simulink model "Speedmeter"  (R2019b)
settings: Solver=FixedStepDiscrete  StartTime=0.0  StopTime=5  FixedStep=0.01  RelTol=1e-3
undefined symbols (not defined in the file or in its folder): Const16_0, Const16_2, Const16_210, Const16_340, Const16_350, Const16_4, Const8_0, Const8_1, Const8_2, Const8_4, ConstFL_00879, ConstFL_01, ConstFL_03516, ConstFL_1_6093, STEP_TIME
libraries: simulink x1
(part 1 of 2)
Description:
  | Integrated model for MBD SWC SpeedMeter
settings Model: DataTypeOverride=Single  ModifiedByFormat=TATA ELXSI LTD  Creator=TATA ELXSI LTD  LastModifiedBy=TATA ELXSI LTD
settings ConfigSet: Description=Test1
settings DataIOCC: LimitDataPoints=on  SaveFormat=StructureWithTime  ReturnWorkspaceOutputs=off
settings OptimizationCC: LifeSpan=inf
settings DebuggingCC: UnderspecifiedInitializationDetection=Classic  MergeDetectMultiDrivingBlocksExec=none  SolverPrmCheckMsg=warning  InheritedTsInSrcMsg=none  ParameterPrecisionLossMsg=none  FcnCallInpInsideContextMsg=warning  StateNameClashWarn=warning  SFUnexpectedBacktrackingDiag=warning  SFNoUnconditionalDefaultTransitionDiag=warning  SFExecutionAtInitializationDiag=none
settings HardwareCC: ProdBitPerPointer=32  ProdBitPerSizeT=32  ProdBitPerPtrDiffT=32  ProdLargestAtomicFloat=None  ProdWordSize=32  ProdHWDeviceType=Generic->32-bit x86 compatible
settings ModelReferenceCC: PropagateSignalLabelsOutOfModel=off
settings RTWCC: Description=Generic Real-Time Target
settings CodeAppCC: StateflowObjectComments=on
settings GRTTargetCC: TargetLangStandard=C89/C90 (ANSI)  CombineOutputUpdateFcns=off  GRTInterface=on
settings ConfigComp: DVMaxTestCaseSteps=500  DVTestSuiteOptimization=CombinedObjectives (Nonlinear Extended)  DVDetectDeadLogic=on  DVDetectActiveLogic=on  DVDetectOutOfBounds=on

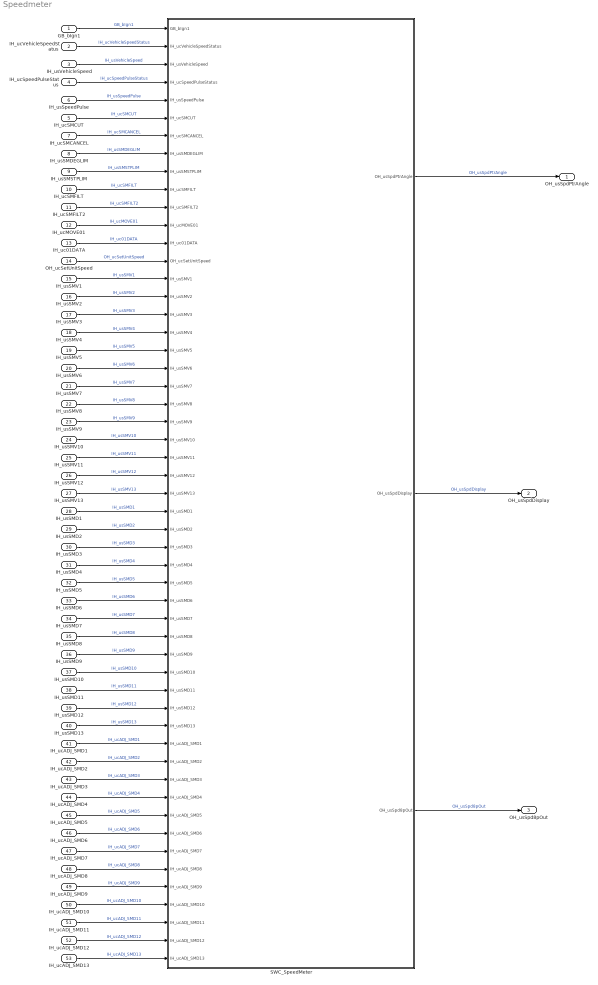
== system Speedmeter ==
  GB_bIgn1 : Inport  OutMin=0  OutMax=1  OutDataTypeStr=uint8  SampleTime=STEP_TIME
  IH_ucVehicleSpeedStatus : Inport  Port=2  OutMin=0  OutMax=3  OutDataTypeStr=fixdt(0,8,1,0)  SampleTime=STEP_TIME
  IH_usVehicleSpeed : Inport  Port=3  OutMin=0  OutMax=655.35  OutDataTypeStr=fixdt(0,16,0.01,0)  SampleTime=STEP_TIME
  IH_ucSpeedPulseStatus : Inport  Port=4  OutMin=0  OutMax=3  OutDataTypeStr=fixdt(0,8,1,0)  SampleTime=STEP_TIME
  IH_ucSMCUT : Inport  Port=5  OutMin=0  OutMax=3  OutDataTypeStr=fixdt(0,8,1,0)  SampleTime=STEP_TIME
  IH_usSpeedPulse : Inport  Port=6  OutMin=0  OutMax=655.35  OutDataTypeStr=fixdt(0,16,0.01,0)  SampleTime=STEP_TIME
  IH_ucSMCANCEL : Inport  Port=7  OutMin=0  OutMax=10.8996  OutDataTypeStr=fixdt(0,8,0.3516,0)  SampleTime=STEP_TIME
  IH_usSMDEGLIM : Inport  Port=8  OutMin=0  OutMax=359.6868  OutDataTypeStr=fixdt(0,16,0.3516,0)  SampleTime=STEP_TIME
  IH_usSMSTPLIM : Inport  Port=9  OutMin=0  OutMax=5.5377  OutDataTypeStr=fixdt(0,16,0.0879,0)  SampleTime=STEP_TIME
  IH_ucSMFILT : Inport  Port=10  OutMin=0  OutMax=7  OutDataTypeStr=fixdt(0,8,1,0)  SampleTime=STEP_TIME
  IH_ucSMFILT2 : Inport  Port=11  OutMin=0  OutMax=7  OutDataTypeStr=fixdt(0,8,1,0)  SampleTime=STEP_TIME
  IH_ucMOVE01 : Inport  Port=12  OutMin=0  OutMax=3  OutDataTypeStr=fixdt(0,8,1,0)  SampleTime=STEP_TIME
  IH_uc01DATA : Inport  Port=13  OutMin=0  OutMax=1  OutDataTypeStr=fixdt(0,8,1,0)  SampleTime=STEP_TIME
  OH_ucSetUnitSpeed : Inport  Port=14  OutMin=0  OutMax=1  OutDataTypeStr=fixdt(0,8,1,0)  SampleTime=STEP_TIME
  IH_usSMV1 : Inport  Port=15  OutMin=0  OutMax=409.5  OutDataTypeStr=fixdt(0,16,0.1,0)  SampleTime=STEP_TIME
  IH_usSMV2 : Inport  Port=16  OutMin=0  OutMax=409.5  OutDataTypeStr=fixdt(0,16,0.1,0)  SampleTime=STEP_TIME
  IH_usSMV3 : Inport  Port=17  OutMin=0  OutMax=409.5  OutDataTypeStr=fixdt(0,16,0.1,0)  SampleTime=STEP_TIME
  IH_usSMV4 : Inport  Port=18  OutMin=0  OutMax=409.5  OutDataTypeStr=fixdt(0,16,0.1,0)  SampleTime=STEP_TIME
  IH_usSMV5 : Inport  Port=19  OutMin=0  OutMax=409.5  OutDataTypeStr=fixdt(0,16,0.1,0)  SampleTime=STEP_TIME
  IH_usSMV6 : Inport  Port=20  OutMin=0  OutMax=409.5  OutDataTypeStr=fixdt(0,16,0.1,0)  SampleTime=STEP_TIME
  IH_usSMV7 : Inport  Port=21  OutMin=0  OutMax=409.5  OutDataTypeStr=fixdt(0,16,0.1,0)  SampleTime=STEP_TIME
  IH_usSMV8 : Inport  Port=22  OutMin=0  OutMax=409.5  OutDataTypeStr=fixdt(0,16,0.1,0)  SampleTime=STEP_TIME
  IH_usSMV9 : Inport  Port=23  OutMin=0  OutMax=409.5  OutDataTypeStr=fixdt(0,16,0.1,0)  SampleTime=STEP_TIME
  IH_usSMV10 : Inport  Port=24  OutMin=0  OutMax=409.5  OutDataTypeStr=fixdt(0,16,0.1,0)  SampleTime=STEP_TIME
  IH_usSMV11 : Inport  Port=25  OutMin=0  OutMax=409.5  OutDataTypeStr=fixdt(0,16,0.1,0)  SampleTime=STEP_TIME
  IH_usSMV12 : Inport  Port=26  OutMin=0  OutMax=409.5  OutDataTypeStr=fixdt(0,16,0.1,0)  SampleTime=STEP_TIME
  IH_usSMV13 : Inport  Port=27  OutMin=0  OutMax=409.5  OutDataTypeStr=fixdt(0,16,0.1,0)  SampleTime=STEP_TIME
  IH_usSMD1 : Inport  Port=28  OutMin=0  OutMax=359.9505  OutDataTypeStr=fixdt(0,16,0.0879,0)  SampleTime=STEP_TIME
  IH_usSMD2 : Inport  Port=29  OutMin=0  OutMax=359.9505  OutDataTypeStr=fixdt(0,16,0.0879,0)  SampleTime=STEP_TIME
  IH_usSMD3 : Inport  Port=30  OutMin=0  OutMax=359.9505  OutDataTypeStr=fixdt(0,16,0.0879,0)  SampleTime=STEP_TIME
  IH_usSMD4 : Inport  Port=31  OutMin=0  OutMax=359.9505  OutDataTypeStr=fixdt(0,16,0.0879,0)  SampleTime=STEP_TIME
  IH_usSMD5 : Inport  Port=32  OutMin=0  OutMax=359.9505  OutDataTypeStr=fixdt(0,16,0.0879,0)  SampleTime=STEP_TIME
  IH_usSMD6 : Inport  Port=33  OutMin=0  OutMax=359.9505  OutDataTypeStr=fixdt(0,16,0.0879,0)  SampleTime=STEP_TIME
  IH_usSMD7 : Inport  Port=34  OutMin=0  OutMax=359.9505  OutDataTypeStr=fixdt(0,16,0.0879,0)  SampleTime=STEP_TIME
  IH_usSMD8 : Inport  Port=35  OutMin=0  OutMax=359.9505  OutDataTypeStr=fixdt(0,16,0.0879,0)  SampleTime=STEP_TIME
  IH_usSMD9 : Inport  Port=36  OutMin=0  OutMax=359.9505  OutDataTypeStr=fixdt(0,16,0.0879,0)  SampleTime=STEP_TIME
  IH_usSMD10 : Inport  Port=37  OutMin=0  OutMax=359.9505  OutDataTypeStr=fixdt(0,16,0.0879,0)  SampleTime=STEP_TIME
  IH_usSMD11 : Inport  Port=38  OutMin=0  OutMax=359.9505  OutDataTypeStr=fixdt(0,16,0.0879,0)  SampleTime=STEP_TIME
  IH_usSMD12 : Inport  Port=39  OutMin=0  OutMax=359.9505  OutDataTypeStr=fixdt(0,16,0.0879,0)  SampleTime=STEP_TIME
  IH_usSMD13 : Inport  Port=40  OutMin=0  OutMax=359.9505  OutDataTypeStr=fixdt(0,16,0.0879,0)  SampleTime=STEP_TIME
  IH_ucADJ_SMD1 : Inport  Port=41  OutMin=0  OutMax=22.4145  OutDataTypeStr=fixdt(0,8,0.0879,0)  SampleTime=STEP_TIME
  IH_ucADJ_SMD2 : Inport  Port=42  OutMin=0  OutMax=22.4145  OutDataTypeStr=fixdt(0,8,0.0879,0)  SampleTime=STEP_TIME
  IH_ucADJ_SMD3 : Inport  Port=43  OutMin=0  OutMax=22.4145  OutDataTypeStr=fixdt(0,8,0.0879,0)  SampleTime=STEP_TIME
  IH_ucADJ_SMD4 : Inport  Port=44  OutMin=0  OutMax=22.4145  OutDataTypeStr=fixdt(0,8,0.0879,0)  SampleTime=STEP_TIME
  IH_ucADJ_SMD5 : Inport  Port=45  OutMin=0  OutMax=22.4145  OutDataTypeStr=fixdt(0,8,0.0879,0)  SampleTime=STEP_TIME
  IH_ucADJ_SMD6 : Inport  Port=46  OutMin=0  OutMax=22.4145  OutDataTypeStr=fixdt(0,8,0.0879,0)  SampleTime=STEP_TIME
  IH_ucADJ_SMD7 : Inport  Port=47  OutMin=0  OutMax=22.4145  OutDataTypeStr=fixdt(0,8,0.0879,0)  SampleTime=STEP_TIME
  IH_ucADJ_SMD8 : Inport  Port=48  OutMin=0  OutMax=22.4145  OutDataTypeStr=fixdt(0,8,0.0879,0)  SampleTime=STEP_TIME
  IH_ucADJ_SMD9 : Inport  Port=49  OutMin=0  OutMax=22.4145  OutDataTypeStr=fixdt(0,8,0.0879,0)  SampleTime=STEP_TIME
  IH_ucADJ_SMD10 : Inport  Port=50  OutMin=0  OutMax=22.4145  OutDataTypeStr=fixdt(0,8,0.0879,0)  SampleTime=STEP_TIME
  IH_ucADJ_SMD11 : Inport  Port=51  OutMin=0  OutMax=22.4145  OutDataTypeStr=fixdt(0,8,0.0879,0)  SampleTime=STEP_TIME
  IH_ucADJ_SMD12 : Inport  Port=52  OutMin=0  OutMax=22.4145  OutDataTypeStr=fixdt(0,8,0.0879,0)  SampleTime=STEP_TIME
  IH_ucADJ_SMD13 : Inport  Port=53  OutMin=0  OutMax=22.4145  OutDataTypeStr=fixdt(0,8,0.0879,0)  SampleTime=STEP_TIME
  SWC_SpeedMeter : Subsystem  LoadFcn=set_param('Speedmeter', 'DataTypeOverride','Single')  TreatAsAtomicUnit=on
  OH_usSpdPtrAngle : Outport  OutMin=0  OutMax=4095  OutDataTypeStr=fixdt(0,16,0.0879,0)  SampleTime=STEP_TIME  VectorParamsAs1DForOutWhenUnconnected=off
  OH_usSpdDisplay : Outport  Port=2  OutDataTypeStr=fixdt(0,16,1,0)  SampleTime=STEP_TIME  VectorParamsAs1DForOutWhenUnconnected=off
  OH_usSpd8pOut : Outport  Port=3  OutMin=0  OutMax=655.34  OutDataTypeStr=fixdt(0,16,0.01,0)  SampleTime=STEP_TIME  VectorParamsAs1DForOutWhenUnconnected=off
  wires:
  IH_ucVehicleSpeedStatus/1 -> SWC_SpeedMeter/2(IH_ucVehicleSpeedStatus)  "IH_ucVehicleSpeedStatus"
  IH_usSMV12/1 -> SWC_SpeedMeter/26(IH_usSMV12)  "IH_usSMV12"
  GB_bIgn1/1 -> SWC_SpeedMeter/1(GB_bIgn1)  "GB_bIgn1"
  IH_ucADJ_SMD6/1 -> SWC_SpeedMeter/46(IH_ucADJ_SMD6)  "IH_ucADJ_SMD6"
  IH_ucADJ_SMD7/1 -> SWC_SpeedMeter/47(IH_ucADJ_SMD7)  "IH_ucADJ_SMD7"
  IH_uc01DATA/1 -> SWC_SpeedMeter/13(IH_uc01DATA)  "IH_uc01DATA"
  IH_ucADJ_SMD12/1 -> SWC_SpeedMeter/52(IH_ucADJ_SMD12)  "IH_ucADJ_SMD12"
  IH_ucADJ_SMD13/1 -> SWC_SpeedMeter/53(IH_ucADJ_SMD13)  "IH_ucADJ_SMD13"
  IH_usVehicleSpeed/1 -> SWC_SpeedMeter/3(IH_usVehicleSpeed)  "IH_usVehicleSpeed"
  IH_ucADJ_SMD11/1 -> SWC_SpeedMeter/51(IH_ucADJ_SMD11)  "IH_ucADJ_SMD11"
  IH_ucADJ_SMD8/1 -> SWC_SpeedMeter/48(IH_ucADJ_SMD8)  "IH_ucADJ_SMD8"
  IH_usSMD9/1 -> SWC_SpeedMeter/36(IH_usSMD9)  "IH_usSMD9"
  IH_usSMD11/1 -> SWC_SpeedMeter/38(IH_usSMD11)  "IH_usSMD11"
  IH_usSMV2/1 -> SWC_SpeedMeter/16(IH_usSMV2)  "IH_usSMV2"
  IH_ucADJ_SMD3/1 -> SWC_SpeedMeter/43(IH_ucADJ_SMD3)  "IH_ucADJ_SMD3"
  IH_usSMD10/1 -> SWC_SpeedMeter/37(IH_usSMD10)  "IH_usSMD10"
  IH_usSMD3/1 -> SWC_SpeedMeter/30(IH_usSMD3)  "IH_usSMD3"
  IH_usSMD13/1 -> SWC_SpeedMeter/40(IH_usSMD13)  "IH_usSMD13"
  OH_ucSetUnitSpeed/1 -> SWC_SpeedMeter/14(OH_ucSetUnitSpeed)  "OH_ucSetUnitSpeed"
  IH_usSMDEGLIM/1 -> SWC_SpeedMeter/8(IH_usSMDEGLIM)  "IH_usSMDEGLIM"
  IH_usSMV13/1 -> SWC_SpeedMeter/27(IH_usSMV13)  "IH_usSMV13"
  IH_usSpeedPulse/1 -> SWC_SpeedMeter/5(IH_usSpeedPulse)  "IH_usSpeedPulse"
  IH_ucADJ_SMD5/1 -> SWC_SpeedMeter/45(IH_ucADJ_SMD5)  "IH_ucADJ_SMD5"
  IH_usSMD5/1 -> SWC_SpeedMeter/32(IH_usSMD5)  "IH_usSMD5"
  IH_ucSMCUT/1 -> SWC_SpeedMeter/6(IH_ucSMCUT)  "IH_ucSMCUT"
  IH_ucSMFILT2/1 -> SWC_SpeedMeter/11(IH_ucSMFILT2)  "IH_ucSMFILT2"
  IH_ucADJ_SMD2/1 -> SWC_SpeedMeter/42(IH_ucADJ_SMD2)  "IH_ucADJ_SMD2"
  IH_usSMD2/1 -> SWC_SpeedMeter/29(IH_usSMD2)  "IH_usSMD2"
  IH_usSMV9/1 -> SWC_SpeedMeter/23(IH_usSMV9)  "IH_usSMV9"
  IH_usSMV8/1 -> SWC_SpeedMeter/22(IH_usSMV8)  "IH_usSMV8"
  IH_usSMD4/1 -> SWC_SpeedMeter/31(IH_usSMD4)  "IH_usSMD4"
  IH_ucSpeedPulseStatus/1 -> SWC_SpeedMeter/4(IH_ucSpeedPulseStatus)  "IH_ucSpeedPulseStatus"
  IH_usSMD6/1 -> SWC_SpeedMeter/33(IH_usSMD6)  "IH_usSMD6"
  IH_usSMV7/1 -> SWC_SpeedMeter/21(IH_usSMV7)  "IH_usSMV7"
  IH_ucADJ_SMD4/1 -> SWC_SpeedMeter/44(IH_ucADJ_SMD4)  "IH_ucADJ_SMD4"
  IH_usSMSTPLIM/1 -> SWC_SpeedMeter/9(IH_usSMSTPLIM)  "IH_usSMSTPLIM"
  IH_usSMD8/1 -> SWC_SpeedMeter/35(IH_usSMD8)  "IH_usSMD8"
  IH_ucADJ_SMD9/1 -> SWC_SpeedMeter/49(IH_ucADJ_SMD9)  "IH_ucADJ_SMD9"
  IH_usSMV5/1 -> SWC_SpeedMeter/19(IH_usSMV5)  "IH_usSMV5"
  IH_usSMD12/1 -> SWC_SpeedMeter/39(IH_usSMD12)  "IH_usSMD12"
  IH_ucSMFILT/1 -> SWC_SpeedMeter/10(IH_ucSMFILT)  "IH_ucSMFILT"
  IH_usSMD1/1 -> SWC_SpeedMeter/28(IH_usSMD1)  "IH_usSMD1"
  IH_usSMV10/1 -> SWC_SpeedMeter/24(IH_usSMV10)  "IH_usSMV10"
  IH_usSMV3/1 -> SWC_SpeedMeter/17(IH_usSMV3)  "IH_usSMV3"
  IH_ucMOVE01/1 -> SWC_SpeedMeter/12(IH_ucMOVE01)  "IH_ucMOVE01"
  IH_ucADJ_SMD10/1 -> SWC_SpeedMeter/50(IH_ucADJ_SMD10)  "IH_ucADJ_SMD10"
  IH_usSMV1/1 -> SWC_SpeedMeter/15(IH_usSMV1)  "IH_usSMV1"
  IH_usSMV4/1 -> SWC_SpeedMeter/18(IH_usSMV4)  "IH_usSMV4"
  IH_usSMV6/1 -> SWC_SpeedMeter/20(IH_usSMV6)  "IH_usSMV6"
  IH_usSMV11/1 -> SWC_SpeedMeter/25(IH_usSMV11)  "IH_usSMV11"
  IH_ucADJ_SMD1/1 -> SWC_SpeedMeter/41(IH_ucADJ_SMD1)  "IH_ucADJ_SMD1"
  IH_ucSMCANCEL/1 -> SWC_SpeedMeter/7(IH_ucSMCANCEL)  "IH_ucSMCANCEL"
  IH_usSMD7/1 -> SWC_SpeedMeter/34(IH_usSMD7)  "IH_usSMD7"
  SWC_SpeedMeter/3(OH_usSpd8pOut) -> OH_usSpd8pOut/1  "OH_usSpd8pOut"
  SWC_SpeedMeter/1(OH_usSpdPtrAngle) -> OH_usSpdPtrAngle/1  "OH_usSpdPtrAngle"
  SWC_SpeedMeter/2(OH_usSpdDisplay) -> OH_usSpdDisplay/1  "OH_usSpdDisplay"

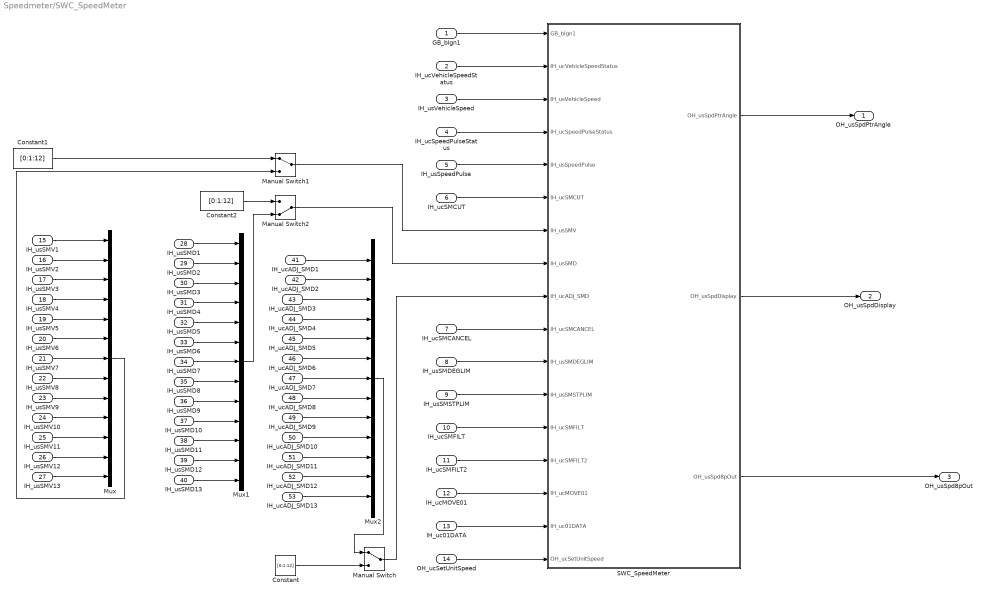
== system Speedmeter/SWC_SpeedMeter ==
  GB_bIgn1 : Inport  SampleTime=STEP_TIME
  IH_ucVehicleSpeedStatus : Inport  Port=2  OutDataTypeStr=fixdt(0,8,1,0)  SampleTime=STEP_TIME
  IH_usVehicleSpeed : Inport  Port=3  OutDataTypeStr=fixdt(0,16,0.01,0)  SampleTime=STEP_TIME
  IH_ucSpeedPulseStatus : Inport  Port=4  OutDataTypeStr=fixdt(0,8,1,0)  SampleTime=STEP_TIME
  IH_usSpeedPulse : Inport  Port=5  OutDataTypeStr=fixdt(0,16,0.01,0)  SampleTime=STEP_TIME
  IH_ucSMCUT : Inport  Port=6  OutDataTypeStr=fixdt(0,8,1,0)  SampleTime=STEP_TIME
  IH_ucSMCANCEL : Inport  Port=7  SampleTime=STEP_TIME
  IH_usSMDEGLIM : Inport  Port=8  SampleTime=STEP_TIME
  IH_usSMSTPLIM : Inport  Port=9  SampleTime=STEP_TIME
  IH_ucSMFILT : Inport  Port=10  OutDataTypeStr=fixdt(0,8,1,0)  SampleTime=STEP_TIME
  IH_ucSMFILT2 : Inport  Port=11  OutDataTypeStr=fixdt(0,8,1,0)  SampleTime=STEP_TIME
  IH_ucMOVE01 : Inport  Port=12  OutDataTypeStr=fixdt(0,8,1,0)  SampleTime=STEP_TIME
  IH_uc01DATA : Inport  Port=13  OutDataTypeStr=fixdt(0,8,1,0)  SampleTime=STEP_TIME
  OH_ucSetUnitSpeed : Inport  Port=14  OutDataTypeStr=fixdt(0,8,1,0)  SampleTime=STEP_TIME
  IH_usSMV1 : Inport  Port=15  SampleTime=STEP_TIME
  IH_usSMV2 : Inport  Port=16  SampleTime=STEP_TIME
  IH_usSMV3 : Inport  Port=17  SampleTime=STEP_TIME
  IH_usSMV4 : Inport  Port=18  SampleTime=STEP_TIME
  IH_usSMV5 : Inport  Port=19  SampleTime=STEP_TIME
  IH_usSMV6 : Inport  Port=20  SampleTime=STEP_TIME
  IH_usSMV7 : Inport  Port=21  SampleTime=STEP_TIME
  IH_usSMV8 : Inport  Port=22  SampleTime=STEP_TIME
  IH_usSMV9 : Inport  Port=23  SampleTime=STEP_TIME
  IH_usSMV10 : Inport  Port=24  SampleTime=STEP_TIME
  IH_usSMV11 : Inport  Port=25  SampleTime=STEP_TIME
  IH_usSMV12 : Inport  Port=26  SampleTime=STEP_TIME
  IH_usSMV13 : Inport  Port=27  SampleTime=STEP_TIME
  IH_usSMD1 : Inport  Port=28  SampleTime=STEP_TIME
  IH_usSMD2 : Inport  Port=29  SampleTime=STEP_TIME
  IH_usSMD3 : Inport  Port=30  SampleTime=STEP_TIME
  IH_usSMD4 : Inport  Port=31  SampleTime=STEP_TIME
  IH_usSMD5 : Inport  Port=32  SampleTime=STEP_TIME
  IH_usSMD6 : Inport  Port=33  SampleTime=STEP_TIME
  IH_usSMD7 : Inport  Port=34  SampleTime=STEP_TIME
  IH_usSMD8 : Inport  Port=35  SampleTime=STEP_TIME
  IH_usSMD9 : Inport  Port=36  SampleTime=STEP_TIME
  IH_usSMD10 : Inport  Port=37  SampleTime=STEP_TIME
  IH_usSMD11 : Inport  Port=38  SampleTime=STEP_TIME
  IH_usSMD12 : Inport  Port=39  SampleTime=STEP_TIME
  IH_usSMD13 : Inport  Port=40  SampleTime=STEP_TIME
  IH_ucADJ_SMD1 : Inport  Port=41  SampleTime=STEP_TIME
  IH_ucADJ_SMD2 : Inport  Port=42  SampleTime=STEP_TIME
  IH_ucADJ_SMD3 : Inport  Port=43  SampleTime=STEP_TIME
  IH_ucADJ_SMD4 : Inport  Port=44  SampleTime=STEP_TIME
  IH_ucADJ_SMD5 : Inport  Port=45  SampleTime=STEP_TIME
  IH_ucADJ_SMD6 : Inport  Port=46  SampleTime=STEP_TIME
  IH_ucADJ_SMD7 : Inport  Port=47  SampleTime=STEP_TIME
  IH_ucADJ_SMD8 : Inport  Port=48  SampleTime=STEP_TIME
  IH_ucADJ_SMD9 : Inport  Port=49  SampleTime=STEP_TIME
  IH_ucADJ_SMD10 : Inport  Port=50  SampleTime=STEP_TIME
  IH_ucADJ_SMD11 : Inport  Port=51  SampleTime=STEP_TIME
  IH_ucADJ_SMD12 : Inport  Port=52  SampleTime=STEP_TIME
  IH_ucADJ_SMD13 : Inport  Port=53  SampleTime=STEP_TIME
  Constant : Constant  Value=[0:1:12]  OutDataTypeStr=fixdt(0,8,0.0879,0)
  Constant1 : Constant  Value=[0:1:12]  OutDataTypeStr=fixdt(0,16,0.1,0)
  Constant2 : Constant  Value=[0:1:12]  OutDataTypeStr=fixdt(0,16,0.0879,0)
  Manual Switch : ManualSwitch
  Manual Switch1 : ManualSwitch
  Manual Switch2 : ManualSwitch  CurrentSetting=0
  Mux : Mux  Inputs=13
  Mux1 : Mux  Inputs=13
  Mux2 : Mux  Inputs=13
  SWC_SpeedMeter : Subsystem  TreatAsAtomicUnit=on
  OH_usSpdPtrAngle : Outport  OutMin=0  OutMax=4095  OutDataTypeStr=fixdt(0,16,0.0879,0)  SampleTime=STEP_TIME  VectorParamsAs1DForOutWhenUnconnected=off
  OH_usSpdDisplay : Outport  Port=2  SampleTime=STEP_TIME  VectorParamsAs1DForOutWhenUnconnected=off
  OH_usSpd8pOut : Outport  Port=3  OutMin=0  OutMax=655.34  OutDataTypeStr=fixdt(0,16,0.01,0)  SampleTime=STEP_TIME  VectorParamsAs1DForOutWhenUnconnected=off
  wires:
  IH_ucADJ_SMD3/1 -> Mux2/3
  Mux1/1 -> Manual Switch2/2
  IH_ucADJ_SMD4/1 -> Mux2/4
  IH_ucADJ_SMD10/1 -> Mux2/10
  Constant1/1 -> Manual Switch1/1
  IH_usSMV11/1 -> Mux/11
  IH_ucADJ_SMD2/1 -> Mux2/2
  IH_ucADJ_SMD7/1 -> Mux2/7
  IH_usSMV12/1 -> Mux/12
  IH_usSMV3/1 -> Mux/3
  IH_usSMD6/1 -> Mux1/6
  Manual Switch/1 -> SWC_SpeedMeter/9(IH_ucADJ_SMD)
  IH_usSMD11/1 -> Mux1/11
  Manual Switch2/1 -> SWC_SpeedMeter/8(IH_usSMD)
  IH_ucADJ_SMD8/1 -> Mux2/8
  IH_ucADJ_SMD11/1 -> Mux2/11
  IH_usSMD1/1 -> Mux1/1
  IH_usSMD12/1 -> Mux1/12
  IH_ucADJ_SMD5/1 -> Mux2/5
  IH_ucSMCUT/1 -> SWC_SpeedMeter/6(IH_ucSMCUT)
  IH_ucADJ_SMD13/1 -> Mux2/13
  Mux2/1 -> Manual Switch/1
  IH_ucADJ_SMD1/1 -> Mux2/1
  IH_ucADJ_SMD6/1 -> Mux2/6
  Constant/1 -> Manual Switch/2
  IH_ucADJ_SMD12/1 -> Mux2/12
  IH_ucSMFILT/1 -> SWC_SpeedMeter/13(IH_ucSMFILT)
  IH_usSMV2/1 -> Mux/2
  IH_usVehicleSpeed/1 -> SWC_SpeedMeter/3(IH_usVehicleSpeed)
  IH_ucADJ_SMD9/1 -> Mux2/9
  IH_usSMD7/1 -> Mux1/7
  IH_usSMD9/1 -> Mux1/9
  IH_usSpeedPulse/1 -> SWC_SpeedMeter/5(IH_usSpeedPulse)
  IH_ucSMCANCEL/1 -> SWC_SpeedMeter/10(IH_ucSMCANCEL)
  SWC_SpeedMeter/2(OH_usSpdDisplay) -> OH_usSpdDisplay/1
  IH_usSMDEGLIM/1 -> SWC_SpeedMeter/11(IH_usSMDEGLIM)
  IH_usSMV4/1 -> Mux/4
  IH_usSMV6/1 -> Mux/6
  IH_ucSMFILT2/1 -> SWC_SpeedMeter/14(IH_ucSMFILT2)
  IH_usSMD2/1 -> Mux1/2
  SWC_SpeedMeter/3(OH_usSpd8pOut) -> OH_usSpd8pOut/1
  IH_usSMSTPLIM/1 -> SWC_SpeedMeter/12(IH_usSMSTPLIM)
  OH_ucSetUnitSpeed/1 -> SWC_SpeedMeter/17(OH_ucSetUnitSpeed)
  IH_usSMD8/1 -> Mux1/8
  SWC_SpeedMeter/1(OH_usSpdPtrAngle) -> OH_usSpdPtrAngle/1
  Manual Switch1/1 -> SWC_SpeedMeter/7(IH_usSMV)
  Constant2/1 -> Manual Switch2/1
  Mux/1 -> Manual Switch1/2
  IH_usSMV13/1 -> Mux/13
  IH_usSMV10/1 -> Mux/10
  IH_usSMV5/1 -> Mux/5
  IH_usSMV7/1 -> Mux/7
  IH_usSMV8/1 -> Mux/8
  IH_usSMV1/1 -> Mux/1
  IH_usSMD5/1 -> Mux1/5
  IH_usSMV9/1 -> Mux/9
  IH_usSMD4/1 -> Mux1/4
  IH_usSMD13/1 -> Mux1/13
  IH_usSMD10/1 -> Mux1/10
  IH_usSMD3/1 -> Mux1/3
  GB_bIgn1/1 -> SWC_SpeedMeter/1(GB_bIgn1)
  IH_ucVehicleSpeedStatus/1 -> SWC_SpeedMeter/2(IH_ucVehicleSpeedStatus)
  IH_ucSpeedPulseStatus/1 -> SWC_SpeedMeter/4(IH_ucSpeedPulseStatus)
  IH_ucMOVE01/1 -> SWC_SpeedMeter/15(IH_ucMOVE01)
  IH_uc01DATA/1 -> SWC_SpeedMeter/16(IH_uc01DATA)

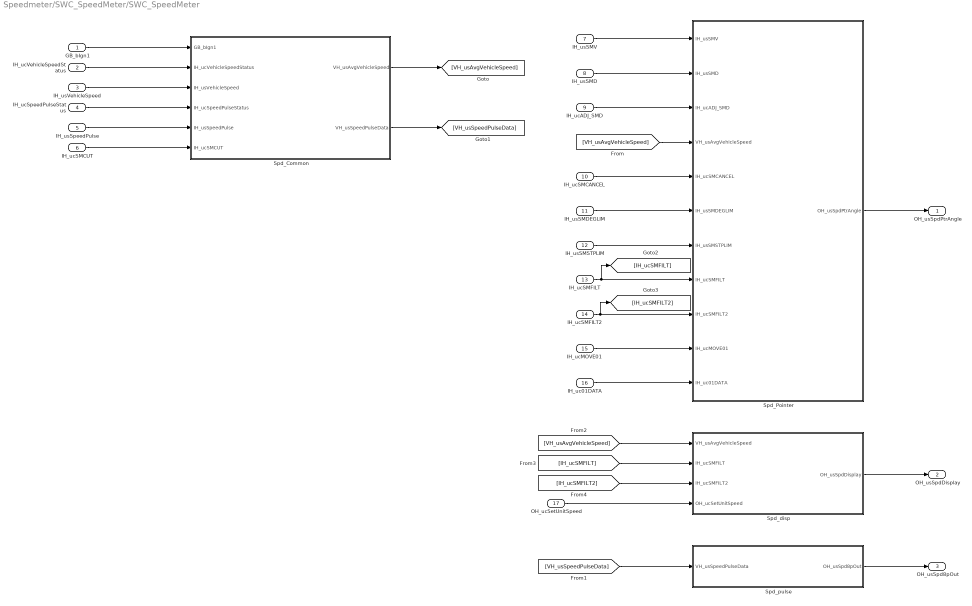
== system Speedmeter/SWC_SpeedMeter/SWC_SpeedMeter ==
  GB_bIgn1 : Inport  SampleTime=STEP_TIME
  IH_ucVehicleSpeedStatus : Inport  Port=2  OutDataTypeStr=fixdt(0,8,1,0)  SampleTime=STEP_TIME
  IH_usVehicleSpeed : Inport  Port=3  OutDataTypeStr=fixdt(0,16,0.01,0)  SampleTime=STEP_TIME
  IH_ucSpeedPulseStatus : Inport  Port=4  OutDataTypeStr=fixdt(0,8,1,0)  SampleTime=STEP_TIME
  IH_usSpeedPulse : Inport  Port=5  OutDataTypeStr=fixdt(0,16,0.01,0)  SampleTime=STEP_TIME
  IH_ucSMCUT : Inport  Port=6  OutDataTypeStr=fixdt(0,8,1,0)  SampleTime=STEP_TIME
  IH_usSMV : Inport  Port=7  SampleTime=STEP_TIME
  IH_usSMD : Inport  Port=8  SampleTime=STEP_TIME
  IH_ucADJ_SMD : Inport  Port=9  SampleTime=STEP_TIME
  IH_ucSMCANCEL : Inport  Port=10  SampleTime=STEP_TIME
  IH_usSMDEGLIM : Inport  Port=11  SampleTime=STEP_TIME
  IH_usSMSTPLIM : Inport  Port=12  SampleTime=STEP_TIME
  IH_ucSMFILT : Inport  Port=13  OutDataTypeStr=fixdt(0,8,1,0)  SampleTime=STEP_TIME
  IH_ucSMFILT2 : Inport  Port=14  OutDataTypeStr=fixdt(0,8,1,0)  SampleTime=STEP_TIME
  IH_ucMOVE01 : Inport  Port=15  OutDataTypeStr=fixdt(0,8,1,0)  SampleTime=STEP_TIME
  IH_uc01DATA : Inport  Port=16  OutDataTypeStr=fixdt(0,8,1,0)  SampleTime=STEP_TIME
  OH_ucSetUnitSpeed : Inport  Port=17  OutDataTypeStr=fixdt(0,8,1,0)  SampleTime=STEP_TIME
  Spd_Common : Subsystem  TreatAsAtomicUnit=on
  Spd_Pointer : Subsystem  TreatAsAtomicUnit=on
  Spd_disp : Subsystem  TreatAsAtomicUnit=on
  Spd_pulse : Subsystem  TreatAsAtomicUnit=on
  OH_usSpdPtrAngle : Outport  SampleTime=STEP_TIME  VectorParamsAs1DForOutWhenUnconnected=off
  OH_usSpdDisplay : Outport  Port=2  SampleTime=STEP_TIME  VectorParamsAs1DForOutWhenUnconnected=off
  OH_usSpd8pOut : Outport  Port=3  OutMin=0  OutMax=655.34  OutDataTypeStr=fixdt(0,16,0.01,0)  SampleTime=STEP_TIME  VectorParamsAs1DForOutWhenUnconnected=off
  wires:
  IH_ucSMCUT/1 -> Spd_Common/6(IH_ucSMCUT)
  Spd_Common/2(VH_usSpeedPulseData) -> [VH_usSpeedPulseData]
  IH_usVehicleSpeed/1 -> Spd_Common/3(IH_usVehicleSpeed)
  IH_usSpeedPulse/1 -> Spd_Common/5(IH_usSpeedPulse)
  Spd_Common/1(VH_usAvgVehicleSpeed) -> [VH_usAvgVehicleSpeed]
  IH_usSMD/1 -> Spd_Pointer/2(IH_usSMD)
  [VH_usAvgVehicleSpeed] -> Spd_disp/1(VH_usAvgVehicleSpeed)
  Spd_pulse/1(OH_usSpd8pOut) -> OH_usSpd8pOut/1
  IH_ucSMFILT2/1 -> [IH_ucSMFILT2], Spd_Pointer/9(IH_ucSMFILT2)
  IH_usSMV/1 -> Spd_Pointer/1(IH_usSMV)
  [VH_usAvgVehicleSpeed] -> Spd_Pointer/4(VH_usAvgVehicleSpeed)
  IH_usSMSTPLIM/1 -> Spd_Pointer/7(IH_usSMSTPLIM)
  OH_ucSetUnitSpeed/1 -> Spd_disp/4(OH_ucSetUnitSpeed)
  IH_ucADJ_SMD/1 -> Spd_Pointer/3(IH_ucADJ_SMD)
  Spd_Pointer/1(OH_usSpdPtrAngle) -> OH_usSpdPtrAngle/1
  [VH_usSpeedPulseData] -> Spd_pulse/1(VH_usSpeedPulseData)
  IH_usSMDEGLIM/1 -> Spd_Pointer/6(IH_usSMDEGLIM)
  IH_ucSMCANCEL/1 -> Spd_Pointer/5(IH_ucSMCANCEL)
  [IH_ucSMFILT] -> Spd_disp/2(IH_ucSMFILT)
  Spd_disp/1(OH_usSpdDisplay) -> OH_usSpdDisplay/1
  [IH_ucSMFILT2] -> Spd_disp/3(IH_ucSMFILT2)
  IH_ucSMFILT/1 -> Spd_Pointer/8(IH_ucSMFILT), [IH_ucSMFILT]
  GB_bIgn1/1 -> Spd_Common/1(GB_bIgn1)
  IH_ucVehicleSpeedStatus/1 -> Spd_Common/2(IH_ucVehicleSpeedStatus)
  IH_ucSpeedPulseStatus/1 -> Spd_Common/4(IH_ucSpeedPulseStatus)
  IH_ucMOVE01/1 -> Spd_Pointer/10(IH_ucMOVE01)
  IH_uc01DATA/1 -> Spd_Pointer/11(IH_uc01DATA)

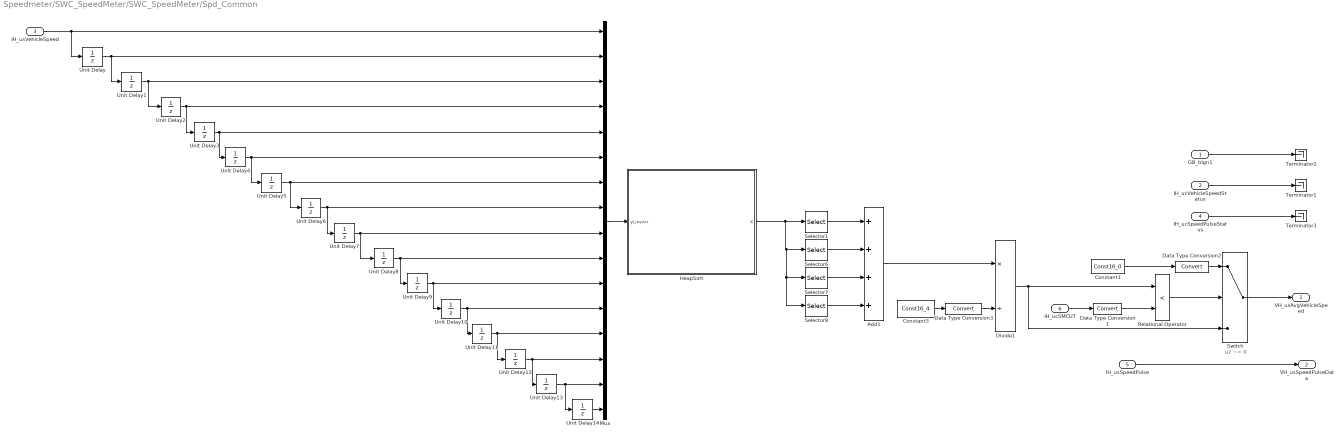
== system Speedmeter/SWC_SpeedMeter/SWC_SpeedMeter/Spd_Common ==
  GB_bIgn1 : Inport  SampleTime=STEP_TIME
  IH_ucVehicleSpeedStatus : Inport  Port=2  OutDataTypeStr=fixdt(0,8,1,0)  SampleTime=STEP_TIME
  IH_usVehicleSpeed : Inport  Port=3  OutDataTypeStr=fixdt(0,16,0.01,0)  SampleTime=STEP_TIME
  IH_ucSpeedPulseStatus : Inport  Port=4  OutDataTypeStr=fixdt(0,8,1,0)  SampleTime=STEP_TIME
  IH_usSpeedPulse : Inport  Port=5  OutDataTypeStr=fixdt(0,16,0.01,0)  SampleTime=STEP_TIME
  IH_ucSMCUT : Inport  Port=6  OutDataTypeStr=fixdt(0,8,1,0)  SampleTime=STEP_TIME
  Add1 : Sum  Inputs=++++  OutDataTypeStr=fixdt(0,32,0.01,0)  InputSameDT=on
  Constant1 : Constant  Value=Const16_0  SampleTime=STEP_TIME
  Constant3 : Constant  Value=Const16_4  OutDataTypeStr=uint16  SampleTime=STEP_TIME
  Data Type Conversion1 : DataTypeConversion
  Data Type Conversion2 : DataTypeConversion
  Data Type Conversion3 : DataTypeConversion
  Divide1 : Product  Inputs=*/  OutDataTypeStr=Inherit: Inherit via back propagation  InputSameDT=on
  HeapSort : Stateflow chart  TreatAsAtomicUnit=on
  Mux : Mux  Inputs=16
  Relational Operator : RelationalOperator  Operator=<  OutDataTypeStr=boolean  RndMeth=Simplest  InputSameDT=on
  Selector1 : Selector  IndexMode=Zero-based  InputPortWidth=16  IndexOptions=Index vector (dialog)  Indices=[6]  OutputSizes=1
  Selector6 : Selector  IndexMode=Zero-based  InputPortWidth=16  IndexOptions=Index vector (dialog)  Indices=[7]  OutputSizes=1
  Selector7 : Selector  IndexMode=Zero-based  InputPortWidth=16  IndexOptions=Index vector (dialog)  Indices=[8]  OutputSizes=1
  Selector8 : Selector  IndexMode=Zero-based  InputPortWidth=16  IndexOptions=Index vector (dialog)  Indices=[9]  OutputSizes=1
  Switch : Switch  Criteria=u2 ~= 0  InputSameDT=on
  Terminator1 : Terminator
  Terminator2 : Terminator
  Terminator3 : Terminator
  Unit Delay{,1..14} (15 alike) : UnitDelay  SampleTime=-1  HasFrameUpgradeWarning=on
  VH_usAvgVehicleSpeed : Outport  OutDataTypeStr=fixdt(0,16,0.01,0)  SampleTime=STEP_TIME  VectorParamsAs1DForOutWhenUnconnected=off
  VH_usSpeedPulseData : Outport  Port=2  OutDataTypeStr=fixdt(0,16,0.01,0)  SampleTime=STEP_TIME  VectorParamsAs1DForOutWhenUnconnected=off
  wires:
  IH_usSpeedPulse/1 -> VH_usSpeedPulseData/1
  Constant1/1 -> Data Type Conversion2/1
  Constant3/1 -> Data Type Conversion3/1
  HeapSort/1(K) -> Selector8/1, Selector7/1, Selector6/1, Selector1/1
  Divide1/1 -> Relational Operator/1, Switch/3
  Add1/1 -> Divide1/1
  Selector7/1 -> Add1/3
  Selector8/1 -> Add1/4
  Selector6/1 -> Add1/2
  Selector1/1 -> Add1/1
  Relational Operator/1 -> Switch/2
  Switch/1 -> VH_usAvgVehicleSpeed/1
  IH_ucSMCUT/1 -> Data Type Conversion1/1
  Data Type Conversion2/1 -> Switch/1
  Data Type Conversion3/1 -> Divide1/2
  Data Type Conversion1/1 -> Relational Operator/2
  IH_usVehicleSpeed/1 -> Unit Delay/1, Mux/1
  Unit Delay14/1 -> Mux/16
  Unit Delay/1 -> Mux/2, Unit Delay1/1
  Unit Delay13/1 -> Unit Delay14/1, Mux/15
  Unit Delay10/1 -> Unit Delay11/1, Mux/12
  Unit Delay7/1 -> Mux/9, Unit Delay8/1
  Unit Delay9/1 -> Unit Delay10/1, Mux/11
  Unit Delay1/1 -> Mux/3, Unit Delay2/1
  Unit Delay12/1 -> Unit Delay13/1, Mux/14
  Unit Delay8/1 -> Mux/10, Unit Delay9/1
  Unit Delay5/1 -> Mux/7, Unit Delay6/1
  Unit Delay4/1 -> Unit Delay5/1, Mux/6
  Unit Delay2/1 -> Mux/4, Unit Delay3/1
  Unit Delay6/1 -> Unit Delay7/1, Mux/8
  Unit Delay11/1 -> Unit Delay12/1, Mux/13
  Unit Delay3/1 -> Unit Delay4/1, Mux/5
  Mux/1 -> HeapSort/1(yLineArr)
  IH_ucSpeedPulseStatus/1 -> Terminator3/1
  IH_ucVehicleSpeedStatus/1 -> Terminator1/1
  GB_bIgn1/1 -> Terminator2/1

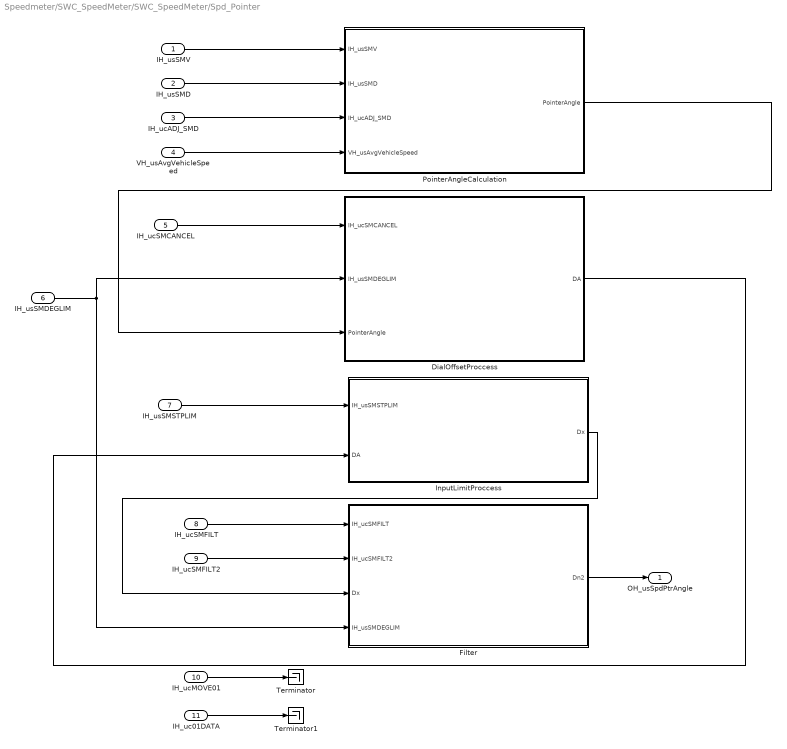
== system Speedmeter/SWC_SpeedMeter/SWC_SpeedMeter/Spd_Pointer ==
  IH_usSMV : Inport  PortDimensions=13  SampleTime=STEP_TIME
  IH_usSMD : Inport  Port=2  PortDimensions=13  SampleTime=STEP_TIME
  IH_ucADJ_SMD : Inport  Port=3  PortDimensions=13  SampleTime=STEP_TIME
  VH_usAvgVehicleSpeed : Inport  Port=4  SampleTime=STEP_TIME
  IH_ucSMCANCEL : Inport  Port=5  SampleTime=STEP_TIME
  IH_usSMDEGLIM : Inport  Port=6  SampleTime=STEP_TIME
  IH_usSMSTPLIM : Inport  Port=7  SampleTime=STEP_TIME
  IH_ucSMFILT : Inport  Port=8  OutDataTypeStr=fixdt(0,8,1,0)  SampleTime=STEP_TIME
  IH_ucSMFILT2 : Inport  Port=9  OutDataTypeStr=fixdt(0,8,1,0)  SampleTime=STEP_TIME
  IH_ucMOVE01 : Inport  Port=10  OutDataTypeStr=fixdt(0,8,1,0)  SampleTime=STEP_TIME
  IH_uc01DATA : Inport  Port=11  OutDataTypeStr=fixdt(0,8,1,0)  SampleTime=STEP_TIME
  DialOffsetProccess : Subsystem  TreatAsAtomicUnit=on
  Filter : Subsystem  TreatAsAtomicUnit=on
  InputLimitProccess : Subsystem  TreatAsAtomicUnit=on
  PointerAngleCalculation : Subsystem  TreatAsAtomicUnit=on
  Terminator : Terminator
  Terminator1 : Terminator
  OH_usSpdPtrAngle : Outport  SampleTime=STEP_TIME  VectorParamsAs1DForOutWhenUnconnected=off
  wires:
  IH_usSMDEGLIM/1 -> Filter/4(IH_usSMDEGLIM), DialOffsetProccess/2(IH_usSMDEGLIM)
  IH_usSMSTPLIM/1 -> InputLimitProccess/1(IH_usSMSTPLIM)
  IH_ucSMCANCEL/1 -> DialOffsetProccess/1(IH_ucSMCANCEL)
  IH_usSMV/1 -> PointerAngleCalculation/1(IH_usSMV)
  DialOffsetProccess/1(DA) -> InputLimitProccess/2(DA)
  IH_ucSMFILT/1 -> Filter/1(IH_ucSMFILT)
  Filter/1(Dn2) -> OH_usSpdPtrAngle/1
  VH_usAvgVehicleSpeed/1 -> PointerAngleCalculation/4(VH_usAvgVehicleSpeed)
  PointerAngleCalculation/1(PointerAngle) -> DialOffsetProccess/3(PointerAngle)
  IH_usSMD/1 -> PointerAngleCalculation/2(IH_usSMD)
  IH_ucADJ_SMD/1 -> PointerAngleCalculation/3(IH_ucADJ_SMD)
  IH_ucSMFILT2/1 -> Filter/2(IH_ucSMFILT2)
  InputLimitProccess/1(Dx) -> Filter/3(Dx)
  IH_uc01DATA/1 -> Terminator1/1
  IH_ucMOVE01/1 -> Terminator/1

== system Speedmeter/SWC_SpeedMeter/SWC_SpeedMeter/Spd_disp ==
  VH_usAvgVehicleSpeed : Inport  SampleTime=STEP_TIME
  IH_ucSMFILT : Inport  Port=2  OutDataTypeStr=fixdt(0,8,1,0)  SampleTime=STEP_TIME
  IH_ucSMFILT2 : Inport  Port=3  OutDataTypeStr=fixdt(0,8,1,0)  SampleTime=STEP_TIME
  OH_ucSetUnitSpeed : Inport  Port=4  OutDataTypeStr=fixdt(0,8,1,0)  SampleTime=STEP_TIME
  Displayfilter : Subsystem  TreatAsAtomicUnit=on
  FilteringProcess : Subsystem  TreatAsAtomicUnit=on
  UnitConversion : Subsystem  TreatAsAtomicUnit=on
  OH_usSpdDisplay : Outport  VectorParamsAs1DForOutWhenUnconnected=off
  wires:
  Displayfilter/1(OH_usSpdDisplay) -> OH_usSpdDisplay/1
  OH_ucSetUnitSpeed/1 -> UnitConversion/1(OH_ucSetUnitSpeed)
  FilteringProcess/1(Dn2) -> [Dn2]
  [Measured_V] -> Displayfilter/1(Measured_V)
  [Dn2] -> UnitConversion/2(Dn2)
  IH_ucSMFILT2/1 -> FilteringProcess/3(IH_ucSMFILT2)
  IH_ucSMFILT/1 -> FilteringProcess/2(IH_ucSMFILT)
  UnitConversion/1(Measured_V) -> [Measured_V]
  VH_usAvgVehicleSpeed/1 -> FilteringProcess/1(VH_usAvgVehicleSpeed)

== system Speedmeter/SWC_SpeedMeter/SWC_SpeedMeter/Spd_pulse ==
  VH_usSpeedPulseData : Inport  OutDataTypeStr=fixdt(0,16,0.01,0)  SampleTime=STEP_TIME
  Constant1 : Constant  Value=Const16_2  OutDataTypeStr=Inherit: Inherit via back propagation  SampleTime=STEP_TIME
  Constant10 : Constant  Value=Const16_350  OutDataTypeStr=Inherit: Inherit via back propagation  SampleTime=STEP_TIME
  Constant11 : Constant  Value=Const16_350  OutDataTypeStr=Inherit: Inherit via back propagation  SampleTime=STEP_TIME
  Constant2 : Constant  Value=Const16_0  OutDataTypeStr=Inherit: Inherit via back propagation  SampleTime=STEP_TIME
  Relational Operator1 : RelationalOperator  Operator=<  OutDataTypeStr=boolean  RndMeth=Simplest  InputSameDT=on
  Relational Operator3 : RelationalOperator  Operator=>  OutDataTypeStr=boolean  RndMeth=Simplest  InputSameDT=on
  Switch1 : Switch  Criteria=u2 ~= 0  InputSameDT=on
  Switch3 : Switch  Criteria=u2 ~= 0  InputSameDT=on
  OH_usSpd8pOut : Outport  OutDataTypeStr=fixdt(0,16,0.01,0)  SampleTime=STEP_TIME  VectorParamsAs1DForOutWhenUnconnected=off
  wires:
  Relational Operator3/1 -> Switch3/2
  VH_usSpeedPulseData/1 -> Relational Operator3/1, Relational Operator1/1, Switch1/3
  Relational Operator1/1 -> Switch1/2
  Switch1/1 -> Switch3/3
  Switch3/1 -> OH_usSpd8pOut/1
  Constant1/1 -> Relational Operator1/2
  Constant2/1 -> Switch1/1
  Constant10/1 -> Relational Operator3/2
  Constant11/1 -> Switch3/1

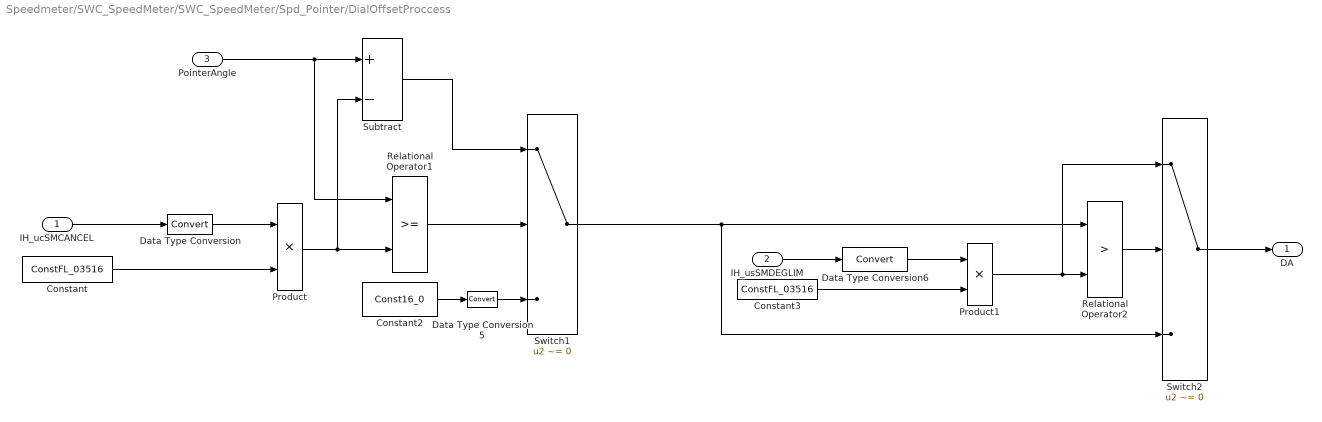
== system Speedmeter/SWC_SpeedMeter/SWC_SpeedMeter/Spd_Pointer/DialOffsetProccess ==
  IH_ucSMCANCEL : Inport  SampleTime=STEP_TIME
  IH_usSMDEGLIM : Inport  Port=2  SampleTime=STEP_TIME
  PointerAngle : Inport  Port=3  OutDataTypeStr=fixdt(1,32,0.0001,0)  SampleTime=STEP_TIME
  Constant : Constant  Value=ConstFL_03516  OutDataTypeStr=fixdt(0,32,0.0001,0)  SampleTime=STEP_TIME
  Constant2 : Constant  Value=Const16_0  SampleTime=STEP_TIME
  Constant3 : Constant  Value=ConstFL_03516  OutDataTypeStr=fixdt(1,32,0.0001,0)  SampleTime=STEP_TIME
  Data Type Conversion : DataTypeConversion
  Data Type Conversion5 : DataTypeConversion
  Data Type Conversion6 : DataTypeConversion
  Product : Product  OutDataTypeStr=fixdt(1,32,0.0001,0)  InputSameDT=on
  Product1 : Product  OutDataTypeStr=fixdt(1,32,0.0001,0)  InputSameDT=on
  Relational Operator1 : RelationalOperator  OutDataTypeStr=boolean  RndMeth=Simplest  InputSameDT=on
  Relational Operator2 : RelationalOperator  Operator=>  OutDataTypeStr=boolean  RndMeth=Simplest  InputSameDT=on
  Subtract : Sum  Inputs=+-  InputSameDT=on
  Switch1 : Switch  Criteria=u2 ~= 0  InputSameDT=on
  Switch2 : Switch  Criteria=u2 ~= 0  InputSameDT=on
  DA : Outport  SampleTime=STEP_TIME  VectorParamsAs1DForOutWhenUnconnected=off
  wires:
  Constant3/1 -> Product1/2
  Subtract/1 -> Switch1/1
  Constant2/1 -> Data Type Conversion5/1
  Product1/1 -> Switch2/1, Relational Operator2/2
  Constant/1 -> Product/2
  Relational Operator1/1 -> Switch1/2
  Product/1 -> Subtract/2, Relational Operator1/2
  PointerAngle/1 -> Subtract/1, Relational Operator1/1
  Data Type Conversion6/1 -> Product1/1
  Data Type Conversion5/1 -> Switch1/3
  Switch1/1 -> Switch2/3, Relational Operator2/1
  Relational Operator2/1 -> Switch2/2
  IH_ucSMCANCEL/1 -> Data Type Conversion/1
  IH_usSMDEGLIM/1 -> Data Type Conversion6/1
  Data Type Conversion/1 -> Product/1
  Switch2/1 -> DA/1

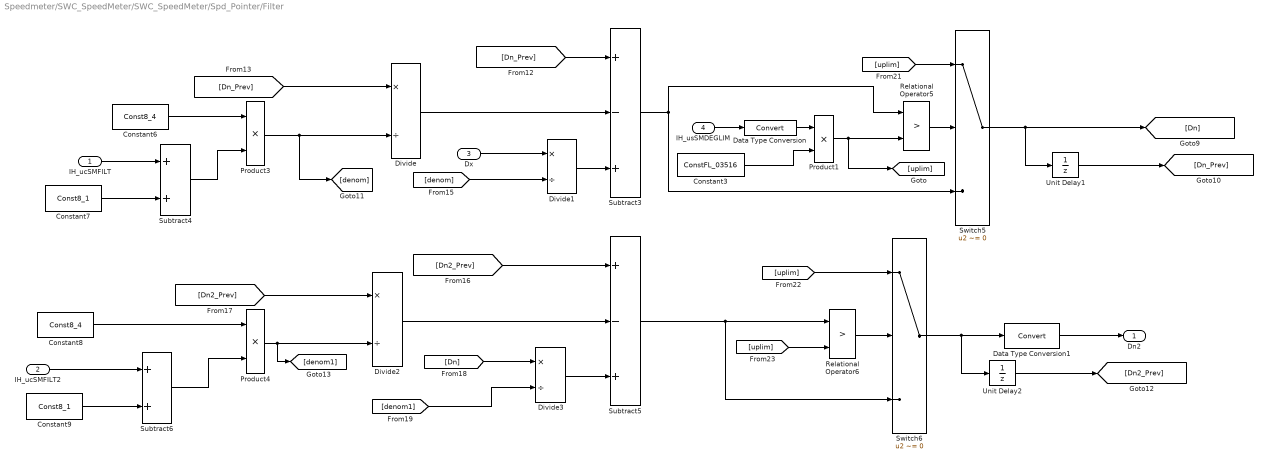
== system Speedmeter/SWC_SpeedMeter/SWC_SpeedMeter/Spd_Pointer/Filter ==
  IH_ucSMFILT : Inport  OutMin=0  OutMax=7  OutDataTypeStr=fixdt(0,8,1,0)  SampleTime=STEP_TIME
  IH_ucSMFILT2 : Inport  Port=2  OutMin=0  OutMax=7  OutDataTypeStr=fixdt(0,8,1,0)  SampleTime=STEP_TIME
  Dx : Inport  Port=3  SampleTime=STEP_TIME
  IH_usSMDEGLIM : Inport  Port=4  OutMin=0  OutMax=1023  SampleTime=STEP_TIME
  Constant3 : Constant  Value=ConstFL_03516  OutDataTypeStr=fixdt(0,32,0.0001,0)  SampleTime=STEP_TIME
  Constant6 : Constant  Value=Const8_4  SampleTime=STEP_TIME
  Constant7 : Constant  Value=Const8_1  OutDataTypeStr=uint8  SampleTime=STEP_TIME
  Constant8 : Constant  Value=Const8_4  SampleTime=STEP_TIME
  Constant9 : Constant  Value=Const8_1  SampleTime=STEP_TIME
  Data Type Conversion : DataTypeConversion
  Data Type Conversion1 : DataTypeConversion  SaturateOnIntegerOverflow=on
  Divide{,1..3} (4 alike) : Product  Inputs=*/  OutDataTypeStr=Inherit: Inherit via back propagation  InputSameDT=on
  Product1 : Product  OutDataTypeStr=fixdt(1,32,0.0001,0)  InputSameDT=on
  Product3 : Product  OutDataTypeStr=fixdt(1,32,0.0001,0)  InputSameDT=on
  Product4 : Product  OutDataTypeStr=fixdt(1,32,0.0001,0)  InputSameDT=on
  Relational Operator5 : RelationalOperator  Operator=>  OutDataTypeStr=boolean  RndMeth=Simplest  InputSameDT=on
  Relational Operator6 : RelationalOperator  Operator=>  OutDataTypeStr=boolean  RndMeth=Simplest  InputSameDT=on
  Subtract3 : Sum  Inputs=+-+  InputSameDT=on
  Subtract4 : Sum  InputSameDT=on
  Subtract5 : Sum  Inputs=+-+  OutDataTypeStr=Inherit: Inherit via back propagation  InputSameDT=on
  Subtract6 : Sum  InputSameDT=on
  Switch5 : Switch  Criteria=u2 ~= 0  InputSameDT=on
  Switch6 : Switch  Criteria=u2 ~= 0  OutDataTypeStr=Inherit: Inherit via back propagation  InputSameDT=on
  Unit Delay1 : UnitDelay  SampleTime=-1  HasFrameUpgradeWarning=on
  Unit Delay2 : UnitDelay  SampleTime=-1  HasFrameUpgradeWarning=on
  Dn2 : Outport  SampleTime=STEP_TIME  VectorParamsAs1DForOutWhenUnconnected=off
  wires:
  Data Type Conversion1/1 -> Dn2/1
  Divide2/1 -> Subtract5/2
  Constant6/1 -> Product3/1
  [uplim] -> Relational Operator6/2
  [Dn2_Prev] -> Subtract5/1
  Subtract4/1 -> Product3/2
  Subtract3/1 -> Relational Operator5/1, Switch5/3
  Product3/1 -> Divide/2, [denom]
  Switch5/1 -> Unit Delay1/1, [Dn]
  Unit Delay1/1 -> [Dn_Prev]
  Product1/1 -> [uplim], Relational Operator5/2
  Product4/1 -> [denom1], Divide2/2
  [Dn] -> Divide3/1
  [denom1] -> Divide3/2
  Constant8/1 -> Product4/1
  IH_ucSMFILT2/1 -> Subtract6/1
  Constant3/1 -> Product1/2
  Dx/1 -> Divide1/1
  Relational Operator5/1 -> Switch5/2
  IH_usSMDEGLIM/1 -> Data Type Conversion/1
  Constant7/1 -> Subtract4/2
  Relational Operator6/1 -> Switch6/2
  [Dn_Prev] -> Subtract3/1
  Data Type Conversion/1 -> Product1/1
  Divide/1 -> Subtract3/2
  [denom] -> Divide1/2
  [uplim] -> Switch6/1
  Unit Delay2/1 -> [Dn2_Prev]
  [Dn_Prev] -> Divide/1
  [Dn2_Prev] -> Divide2/1
  Switch6/1 -> Data Type Conversion1/1, Unit Delay2/1
  Divide3/1 -> Subtract5/3
  [uplim] -> Switch5/1
  Subtract6/1 -> Product4/2
  Constant9/1 -> Subtract6/2
  Subtract5/1 -> Relational Operator6/1, Switch6/3
  IH_ucSMFILT/1 -> Subtract4/1
  Divide1/1 -> Subtract3/3

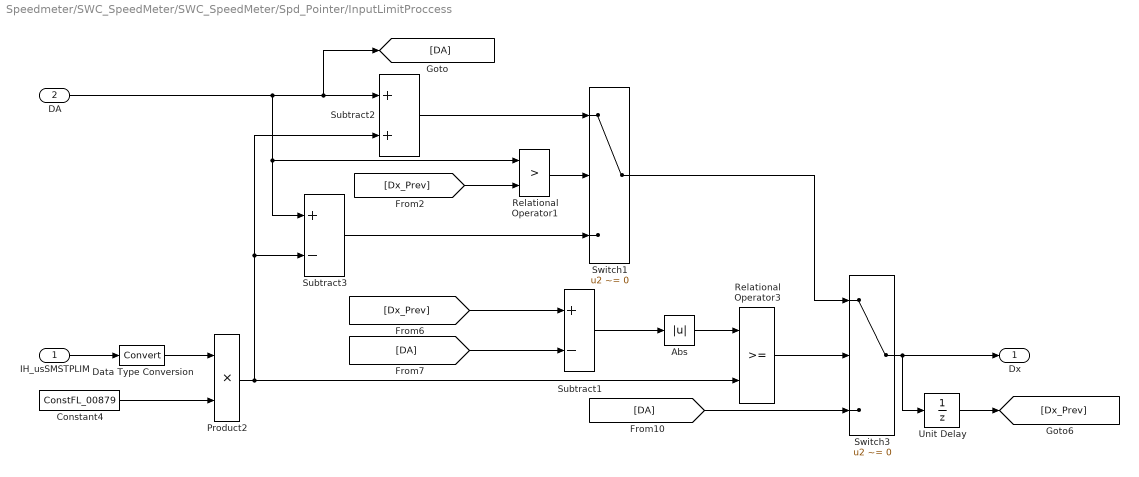
== system Speedmeter/SWC_SpeedMeter/SWC_SpeedMeter/Spd_Pointer/InputLimitProccess ==
  IH_usSMSTPLIM : Inport  SampleTime=STEP_TIME
  DA : Inport  Port=2  SampleTime=STEP_TIME
  Abs : Abs  OutDataTypeStr=fixdt(1,32,0.0001,0)
  Constant4 : Constant  Value=ConstFL_00879  OutDataTypeStr=fixdt(0,32,0.0001,0)  SampleTime=STEP_TIME
  Data Type Conversion : DataTypeConversion
  Product2 : Product  OutDataTypeStr=Inherit: Inherit via back propagation  InputSameDT=on
  Relational Operator1 : RelationalOperator  Operator=>  OutDataTypeStr=boolean  RndMeth=Simplest  InputSameDT=on
  Relational Operator3 : RelationalOperator  OutDataTypeStr=boolean  RndMeth=Simplest  InputSameDT=on
  Subtract1 : Sum  Inputs=+-  InputSameDT=on
  Subtract2 : Sum  InputSameDT=on
  Subtract3 : Sum  Inputs=+-  InputSameDT=on
  Switch1 : Switch  Criteria=u2 ~= 0  OutDataTypeStr=Inherit: Inherit via back propagation  InputSameDT=on
  Switch3 : Switch  Criteria=u2 ~= 0  OutDataTypeStr=Inherit: Inherit via back propagation  InputSameDT=on
  Unit Delay : UnitDelay  SampleTime=-1  HasFrameUpgradeWarning=on
  Dx : Outport  SampleTime=STEP_TIME  VectorParamsAs1DForOutWhenUnconnected=off
  wires:
  Constant4/1 -> Product2/2
  [Dx_Prev] -> Relational Operator1/2
  Subtract3/1 -> Switch1/3
  Switch1/1 -> Switch3/1
  Relational Operator1/1 -> Switch1/2
  Relational Operator3/1 -> Switch3/2
  [DA] -> Subtract1/2
  Subtract2/1 -> Switch1/1
  Subtract1/1 -> Abs/1
  Switch3/1 -> Dx/1, Unit Delay/1
  [DA] -> Switch3/3
  Abs/1 -> Relational Operator3/1
  IH_usSMSTPLIM/1 -> Data Type Conversion/1
  Data Type Conversion/1 -> Product2/1
  Product2/1 -> Relational Operator3/2, Subtract2/2, Subtract3/2
  [Dx_Prev] -> Subtract1/1
  DA/1 -> Subtract3/1, Relational Operator1/1, [DA], Subtract2/1
  Unit Delay/1 -> [Dx_Prev]

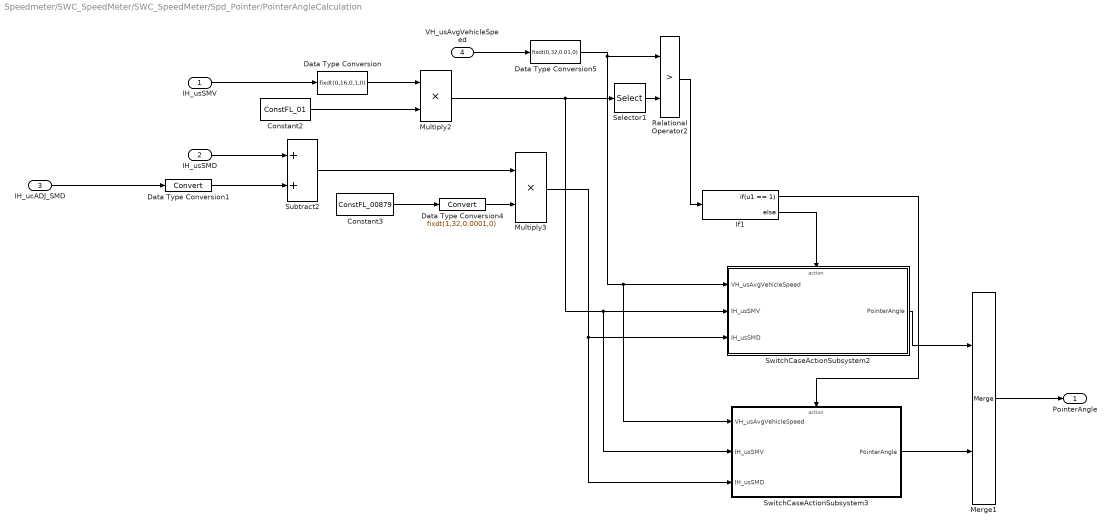
== system Speedmeter/SWC_SpeedMeter/SWC_SpeedMeter/Spd_Pointer/PointerAngleCalculation ==
  IH_usSMV : Inport  SampleTime=STEP_TIME
  IH_usSMD : Inport  Port=2  SampleTime=STEP_TIME
  IH_ucADJ_SMD : Inport  Port=3  SampleTime=STEP_TIME
  VH_usAvgVehicleSpeed : Inport  Port=4  SampleTime=STEP_TIME
  Constant2 : Constant  Value=ConstFL_01  SampleTime=STEP_TIME
  Constant3 : Constant  Value=ConstFL_00879  SampleTime=STEP_TIME
  Data Type Conversion : DataTypeConversion  OutDataTypeStr=fixdt(0,16,0.1,0)
  Data Type Conversion1 : DataTypeConversion
  Data Type Conversion4 : DataTypeConversion  OutDataTypeStr=fixdt(1,32,0.0001,0)
  Data Type Conversion5 : DataTypeConversion  OutDataTypeStr=fixdt(0,32,0.01,0)
  If1 : If  IfExpression=u1 == 1
  Merge1 : Merge  InitialOutput=0
  Multiply2 : Product  OutDataTypeStr=fixdt(0,32,0.01,0)  InputSameDT=on
  Multiply3 : Product  InputSameDT=on  OutDataTypeStr=Inherit: Same as first input
  Relational Operator2 : RelationalOperator  Operator=>  OutDataTypeStr=boolean  RndMeth=Simplest
  Selector1 : Selector  IndexMode=Zero-based  InputPortWidth=13  IndexOptions=Index vector (dialog)  Indices=[12]  OutputSizes=1
  Subtract2 : Sum  OutDataTypeStr=Inherit: Inherit via back propagation  InputSameDT=on
  SwitchCaseActionSubsystem2 : Subsystem  TreatAsAtomicUnit=on
  SwitchCaseActionSubsystem3 : Subsystem  TreatAsAtomicUnit=on
  PointerAngle : Outport  SampleTime=STEP_TIME  VectorParamsAs1DForOutWhenUnconnected=off
  wires:
  Constant2/1 -> Multiply2/2
  Selector1/1 -> Relational Operator2/2
  IH_ucADJ_SMD/1 -> Data Type Conversion1/1
  If1/1 -> SwitchCaseActionSubsystem3/Action
  IH_usSMD/1 -> Subtract2/1
  If1/2 -> SwitchCaseActionSubsystem2/Action
  SwitchCaseActionSubsystem3/1(PointerAngle) -> Merge1/2
  Data Type Conversion4/1 -> Multiply3/2
  Multiply2/1 -> Selector1/1, SwitchCaseActionSubsystem2/2(IH_usSMV), SwitchCaseActionSubsystem3/2(IH_usSMV)
  Merge1/1 -> PointerAngle/1
  Relational Operator2/1 -> If1/1
  Subtract2/1 -> Multiply3/1
  Data Type Conversion5/1 -> SwitchCaseActionSubsystem2/1(VH_usAvgVehicleSpeed), SwitchCaseActionSubsystem3/1(VH_usAvgVehicleSpeed), Relational Operator2/1
  Data Type Conversion/1 -> Multiply2/1
  SwitchCaseActionSubsystem2/1(PointerAngle) -> Merge1/1
  Constant3/1 -> Data Type Conversion4/1
  VH_usAvgVehicleSpeed/1 -> Data Type Conversion5/1
  IH_usSMV/1 -> Data Type Conversion/1
  Multiply3/1 -> SwitchCaseActionSubsystem2/3(IH_usSMD), SwitchCaseActionSubsystem3/3(IH_usSMD)
  Data Type Conversion1/1 -> Subtract2/2

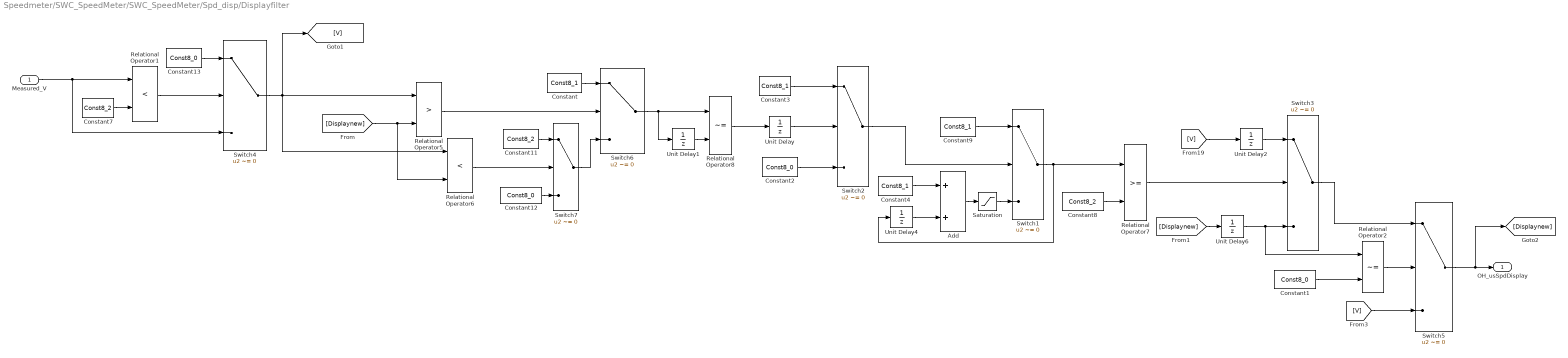
== system Speedmeter/SWC_SpeedMeter/SWC_SpeedMeter/Spd_disp/Displayfilter ==
  Measured_V : Inport  OutDataTypeStr=fixdt(0,16,1,0)
  Add : Sum  InputSameDT=on
  Constant{,3..4,9} (4 alike) : Constant  Value=Const8_1
  Constant1 : Constant  Value=Const8_0  OutDataTypeStr=Inherit: Inherit via back propagation
  Constant11 : Constant  Value=Const8_2
  Constant12 : Constant  Value=Const8_0
  Constant13 : Constant  Value=Const8_0  OutDataTypeStr=Inherit: Inherit via back propagation
  Constant2 : Constant  Value=Const8_0
  Constant7 : Constant  Value=Const8_2  OutDataTypeStr=Inherit: Inherit via back propagation
  Constant8 : Constant  Value=Const8_2
  Relational Operator1 : RelationalOperator  Operator=<  OutDataTypeStr=boolean  RndMeth=Simplest  InputSameDT=on
  Relational Operator2 : RelationalOperator  Operator=~=  OutDataTypeStr=boolean  RndMeth=Simplest  InputSameDT=on
  Relational Operator5 : RelationalOperator  Operator=>  OutDataTypeStr=boolean  RndMeth=Simplest  InputSameDT=on
  Relational Operator6 : RelationalOperator  Operator=<  OutDataTypeStr=boolean  RndMeth=Simplest  InputSameDT=on
  Relational Operator7 : RelationalOperator  OutDataTypeStr=boolean  RndMeth=Simplest  InputSameDT=on
  Relational Operator8 : RelationalOperator  Operator=~=  OutDataTypeStr=boolean  RndMeth=Simplest  InputSameDT=on
  Saturation : Saturate  UpperLimit=3  LowerLimit=1  OutDataTypeStr=uint8
  Switch1 : Switch  Criteria=u2 ~= 0  Threshold=2  InputSameDT=on
  Switch2 : Switch  Criteria=u2 ~= 0  Threshold=2  InputSameDT=on
  Switch3 : Switch  Criteria=u2 ~= 0  OutDataTypeStr=Inherit: Inherit via back propagation  InputSameDT=on
  Switch{4..7} (4 alike) : Switch  Criteria=u2 ~= 0  InputSameDT=on
  Unit Delay{,1..2,4,6} (5 alike) : UnitDelay  SampleTime=-1  HasFrameUpgradeWarning=on
  OH_usSpdDisplay : Outport  OutDataTypeStr=fixdt(0,16,1,0)  VectorParamsAs1DForOutWhenUnconnected=off
  wires:
  [V] -> Unit Delay2/1
  Constant13/1 -> Switch4/1
  Relational Operator7/1 -> Switch3/2
  Relational Operator6/1 -> Switch7/2
  Relational Operator5/1 -> Switch6/2
  [V] -> Switch5/3
  Constant1/1 -> Relational Operator2/2
  Unit Delay2/1 -> Switch3/1
  Saturation/1 -> Switch1/3
  Constant7/1 -> Relational Operator1/2
  Constant9/1 -> Switch1/1
  Switch7/1 -> Switch6/3
  Constant/1 -> Switch6/1
  [Displaynew] -> Unit Delay6/1
  Constant12/1 -> Switch7/3
  Measured_V/1 -> Switch4/3, Relational Operator1/1
  Constant3/1 -> Switch2/1
  Constant11/1 -> Switch7/1
  Switch3/1 -> Switch5/1
  Unit Delay/1 -> Switch2/2
  Add/1 -> Saturation/1
  Constant2/1 -> Switch2/3
  Switch6/1 -> Unit Delay1/1, Relational Operator8/1
  Unit Delay1/1 -> Relational Operator8/2
  Constant4/1 -> Add/1
  Unit Delay6/1 -> Relational Operator2/1, Switch3/3
  Relational Operator1/1 -> Switch4/2
  Switch1/1 -> Relational Operator7/1, Unit Delay4/1
  [Displaynew] -> Relational Operator5/2, Relational Operator6/2
  Constant8/1 -> Relational Operator7/2
  Switch4/1 -> [V], Relational Operator5/1, Relational Operator6/1
  Relational Operator2/1 -> Switch5/2
  Unit Delay4/1 -> Add/2
  Relational Operator8/1 -> Unit Delay/1
  Switch5/1 -> [Displaynew], OH_usSpdDisplay/1
  Switch2/1 -> Switch1/2

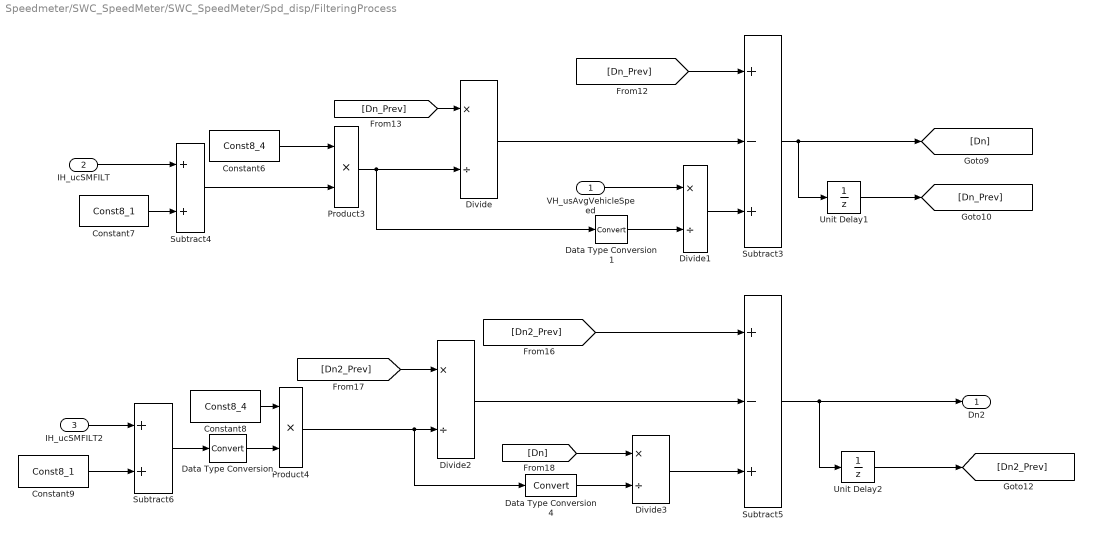
== system Speedmeter/SWC_SpeedMeter/SWC_SpeedMeter/Spd_disp/FilteringProcess ==
  VH_usAvgVehicleSpeed : Inport  SampleTime=STEP_TIME
  IH_ucSMFILT : Inport  Port=2  OutDataTypeStr=fixdt(0,8,1,0)  SampleTime=STEP_TIME
  IH_ucSMFILT2 : Inport  Port=3  OutDataTypeStr=fixdt(0,8,1,0)  SampleTime=STEP_TIME
  Constant6 : Constant  Value=Const8_4  SampleTime=STEP_TIME
  Constant7 : Constant  Value=Const8_1  SampleTime=STEP_TIME
  Constant8 : Constant  Value=Const8_4  SampleTime=STEP_TIME
  Constant9 : Constant  Value=Const8_1  SampleTime=STEP_TIME
  Data Type Conversion : DataTypeConversion
  Data Type Conversion1 : DataTypeConversion
  Data Type Conversion4 : DataTypeConversion
  Divide{,1..3} (4 alike) : Product  Inputs=*/  OutDataTypeStr=fixdt(0,16,0.1,0)  InputSameDT=on
  Product3 : Product  OutDataTypeStr=Inherit: Inherit via back propagation  InputSameDT=on
  Product4 : Product  OutDataTypeStr=Inherit: Inherit via back propagation  InputSameDT=on
  Subtract3 : Sum  Inputs=+-+  InputSameDT=on
  Subtract4 : Sum  InputSameDT=on
  Subtract5 : Sum  Inputs=+-+  InputSameDT=on
  Subtract6 : Sum  OutDataTypeStr=uint16  InputSameDT=on
  Unit Delay1 : UnitDelay  SampleTime=-1  HasFrameUpgradeWarning=on
  Unit Delay2 : UnitDelay  SampleTime=-1  HasFrameUpgradeWarning=on
  Dn2 : Outport  SampleTime=STEP_TIME  VectorParamsAs1DForOutWhenUnconnected=off
  wires:
  Subtract5/1 -> Dn2/1, Unit Delay2/1
  IH_ucSMFILT/1 -> Subtract4/1
  Constant6/1 -> Product3/1
  Divide2/1 -> Subtract5/2
  Divide3/1 -> Subtract5/3
  Product3/1 -> Data Type Conversion1/1, Divide/2
  Subtract4/1 -> Product3/2
  [Dn2_Prev] -> Divide2/1
  Product4/1 -> Data Type Conversion4/1, Divide2/2
  [Dn] -> Divide3/1
  Constant7/1 -> Subtract4/2
  IH_ucSMFILT2/1 -> Subtract6/1
  [Dn_Prev] -> Divide/1
  VH_usAvgVehicleSpeed/1 -> Divide1/1
  Subtract6/1 -> Data Type Conversion/1
  Subtract3/1 -> Unit Delay1/1, [Dn]
  Divide/1 -> Subtract3/2
  Constant8/1 -> Product4/1
  Divide1/1 -> Subtract3/3
  Constant9/1 -> Subtract6/2
  Data Type Conversion/1 -> Product4/2
  Data Type Conversion1/1 -> Divide1/2
  [Dn_Prev] -> Subtract3/1
  Unit Delay1/1 -> [Dn_Prev]
  Data Type Conversion4/1 -> Divide3/2
  [Dn2_Prev] -> Subtract5/1
  Unit Delay2/1 -> [Dn2_Prev]

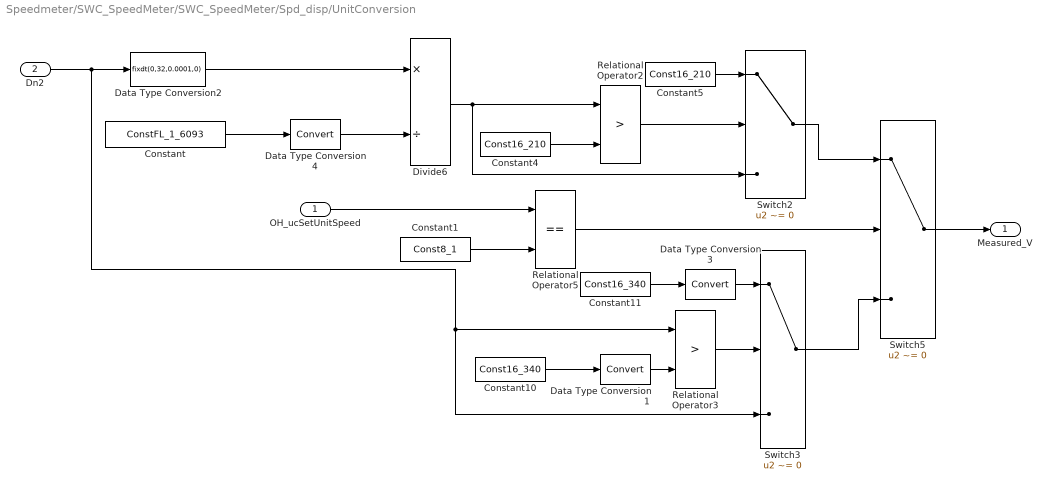
== system Speedmeter/SWC_SpeedMeter/SWC_SpeedMeter/Spd_disp/UnitConversion ==
  OH_ucSetUnitSpeed : Inport  OutDataTypeStr=fixdt(0,8,1,0)  SampleTime=STEP_TIME
  Dn2 : Inport  Port=2  OutDataTypeStr=fixdt(0,16,0.1,0)  SampleTime=STEP_TIME
  Constant : Constant  Value=ConstFL_1_6093  SampleTime=STEP_TIME
  Constant1 : Constant  Value=Const8_1  SampleTime=STEP_TIME
  Constant10 : Constant  Value=Const16_340  SampleTime=STEP_TIME
  Constant11 : Constant  Value=Const16_340  SampleTime=STEP_TIME
  Constant4 : Constant  Value=Const16_210  OutDataTypeStr=Inherit: Inherit via back propagation  SampleTime=STEP_TIME
  Constant5 : Constant  Value=Const16_210  OutDataTypeStr=Inherit: Inherit via back propagation  SampleTime=STEP_TIME
  Data Type Conversion1 : DataTypeConversion
  Data Type Conversion2 : DataTypeConversion  OutDataTypeStr=fixdt(0,32,0.0001,0)
  Data Type Conversion3 : DataTypeConversion
  Data Type Conversion4 : DataTypeConversion
  Divide6 : Product  Inputs=*/  OutDataTypeStr=fixdt(0,16,0.01,0)  InputSameDT=on
  Relational Operator2 : RelationalOperator  Operator=>  OutDataTypeStr=boolean  RndMeth=Simplest  InputSameDT=on
  Relational Operator3 : RelationalOperator  Operator=>  OutDataTypeStr=boolean  RndMeth=Simplest  InputSameDT=on
  Relational Operator5 : RelationalOperator  Operator===  OutDataTypeStr=boolean  RndMeth=Simplest  InputSameDT=on
  Switch2 : Switch  Criteria=u2 ~= 0  OutDataTypeStr=Inherit: Inherit via back propagation  InputSameDT=on
  Switch3 : Switch  Criteria=u2 ~= 0  InputSameDT=on
  Switch5 : Switch  Criteria=u2 ~= 0  OutDataTypeStr=Inherit: Inherit via back propagation  InputSameDT=on
  Measured_V : Outport  OutDataTypeStr=fixdt(0,16,1,0)  SampleTime=STEP_TIME  VectorParamsAs1DForOutWhenUnconnected=off
  wires:
  OH_ucSetUnitSpeed/1 -> Relational Operator5/1
  Dn2/1 -> Relational Operator3/1, Switch3/3, Data Type Conversion2/1
  Constant1/1 -> Relational Operator5/2
  Constant10/1 -> Data Type Conversion1/1
  Constant/1 -> Data Type Conversion4/1
  Relational Operator3/1 -> Switch3/2
  Relational Operator2/1 -> Switch2/2
  Constant11/1 -> Data Type Conversion3/1
  Data Type Conversion1/1 -> Relational Operator3/2
  Divide6/1 -> Relational Operator2/1, Switch2/3
  Constant5/1 -> Switch2/1
  Relational Operator5/1 -> Switch5/2
  Switch3/1 -> Switch5/3
  Switch2/1 -> Switch5/1
  Data Type Conversion2/1 -> Divide6/1
  Switch5/1 -> Measured_V/1
  Constant4/1 -> Relational Operator2/2
  Data Type Conversion3/1 -> Switch3/1
  Data Type Conversion4/1 -> Divide6/2

== system Speedmeter/SWC_SpeedMeter/SWC_SpeedMeter/Spd_Pointer/PointerAngleCalculation/SwitchCaseActionSubsystem2 ==
  VH_usAvgVehicleSpeed : Inport  PortDimensions=1  SampleTime=STEP_TIME
  IH_usSMV : Inport  Port=2  OutMin=0  OutMax=4095  SampleTime=STEP_TIME
  IH_usSMD : Inport  Port=3  OutMin=0  OutMax=4095  SampleTime=STEP_TIME
  Action Port : ActionPort  ActionPortLabel=else { }
  Lookup Table Dynamic : simulink/Lookup Tables/Lookup Table Dynamic  LookUpMeth=Interpolation-Use End Values  OutDataType=fixdt(0,16,0.1,0)  OutScaling=[]  OutDataTypeStr=Inherit: Inherit via back propagation  DoSatur=off
      settings: SourceProductName=Simulink
  PointerAngle : Outport  SampleTime=STEP_TIME  VectorParamsAs1DForOutWhenUnconnected=off
  wires:
  VH_usAvgVehicleSpeed/1 -> Lookup Table Dynamic/1
  IH_usSMV/1 -> Lookup Table Dynamic/2
  Lookup Table Dynamic/1 -> PointerAngle/1
  IH_usSMD/1 -> Lookup Table Dynamic/3
